simulink model "Supervisory_Logic"  (R2023b)
settings: Solver=FixedStepDiscrete  StartTime=0.0  StopTime=10  RelTol=1e-3
model workspace (MAT data in the model file):
  TsModel = 0.1
settings Model: ExtModeTrigDuration=8  Creator=vivekr  LastModifiedBy=vlenzi
settings SolverCC: AlgebraicLoopSolver=TrustRegion
settings DataIOCC: SaveFormat=StructureWithTime  SaveOutput=off  SignalLogging=off  DSMLogging=off  SaveTime=off  SignalLoggingName=logsOut
settings OptimizationCC: DefaultParameterBehavior=Inlined  UseDivisionForNetSlopeComputation=UseDivisionForReciprocalsOfIntegersOnly  ReuseModelBlockBuffer=off  EnhancedBackFolding=on  BooleansAsBitfields=on  PassReuseOutputArgsAs=Individual arguments  ExpressionDepthLimit=2147483647  StateBitsets=on  DataBitsets=on  ZeroExternalMemoryAtStartup=off  NoFixptDivByZeroProtection=on  EfficientFloat2IntCast=on  LifeSpan=1  MaxStackSize=64  SimCompilerOptimization=on  EfficientTunableParamExpr=on
settings DebuggingCC: ReadBeforeWriteMsg=DisableAll  WriteAfterWriteMsg=DisableAll  WriteAfterReadMsg=DisableAll  CheckExecutionContextPreStartOutputMsg=on  ParameterPrecisionLossMsg=none  UnconnectedInputMsg=warning  UnconnectedOutputMsg=warning  UnconnectedLineMsg=warning  UniqueDataStoreMsg=error  AllowSymbolicDim=off  ModelReferenceSymbolNameMessage=none  StateNameClashWarn=warning  StrictBusMsg=ErrorOnBusTreatedAsVector  SymbolicDimsDataTypeCodeGenerationDiagnostic=none  SFUnexpectedBacktrackingDiag=warning  SFNoUnconditionalDefaultTransitionDiag=warning  SFExecutionAtInitializationDiag=none  ArithmeticOperatorsInVariantConditions=warning
settings HardwareCC: TargetHWDeviceType=Generic->32-bit Embedded Processor
settings ModelReferenceCC: EnableRefExpFcnMdlSchedulingChecks=on  CheckModelReferenceTargetMessage=none  PropagateSignalLabelsOutOfModel=off
settings SFSimCC: SimUseLocalCustomCode=off  MATLABDynamicMemAlloc=off
settings RTWCC: Description=Embedded Coder  SystemTargetFile=ert.tlc  TemplateMakefile=ert_default_tmf  GenerateReport=on  RTWVerbose=off  RTWUseLocalCustomCode=off  IncludeHyperlinkInReport=on  PortableWordSizes=on  CodeExecutionProfiling=on  CodeProfilingSaveOptions=AllData  CodeProfilingInstrumentation=coarse  GenerateTraceInfo=on  GenerateTraceReport=on  GenerateTraceReportSl=on  GenerateTraceReportSf=on  GenerateTraceReportEml=on  GenerateCodeMetricsReport=on  DLArmComputeVersion=19.05
settings CodeAppCC: ForceParamTrailComments=on  IgnoreCustomStorageClasses=off  SimulinkDataObjDesc=on  CustomSymbolStrGlobalVar=rt$N$M  CustomSymbolStrType=$N$M  CustomSymbolStrFcn=$N$M$F  CustomSymbolStrMacro=$N$M  InsertBlockDesc=on  StateflowObjectComments=on  InternalIdentifier=Classic
settings ERTTargetCC: UtilityFuncGeneration=Shared location  MultiwordLength=2048  IncludeMdlTerminateFcn=off  CombineSignalStateStructs=on  SupportNonFinite=off  SupportComplex=off  ExtModeStaticAllocSize=2048  ERTCustomFileTemplate=example_file_process.tlc  ERTFilePackagingFormat=CompactWithDataFile  ConvertIfToSwitch=off  SuppressUnreachableDefaultCases=off
settings ConfigComp: CovMetricSettings=dw  CovSaveCumulativeToWorkspaceVar=on  CovSaveSingleToWorkspaceVar=on  CovExternalEMLEnable=off  CovSFcnEnable=off  PLC_TargetIDE=codesys35  PLC_MultiTBSigbuilderTimeRange=off  PLC_GenerateReusableCode=on  PLC_FoldFBCallOutputVar=on  PLC_RemoveUnusedSSMethodCallArguments=on  PLC_FBUseSubsystemInstanceName=on  PLC_UseCallOutputArgSyntax=off  PLC_EnableUnsignedAndDoubleTypes=off  PLC_EnableUDTSplitting=off  PLC_MaxFieldsInUDT=500  PLC_GenerateEnumSymbolicName=on  PLC_GenerateEnumCastFunction=on  PLC_InlineEnumCastFunction=on  PLC_GenerateWebView=on

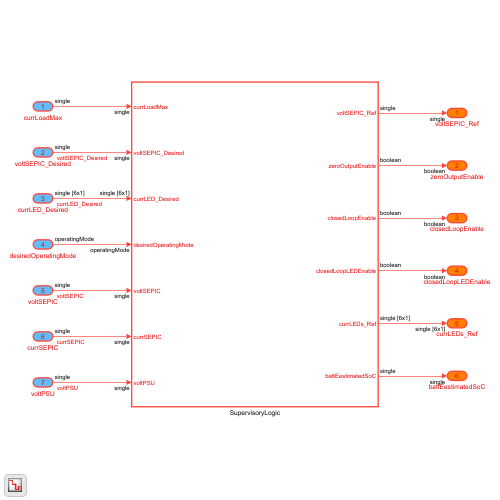
[thumbnail: Simulink's stored preview of the top-level diagram]
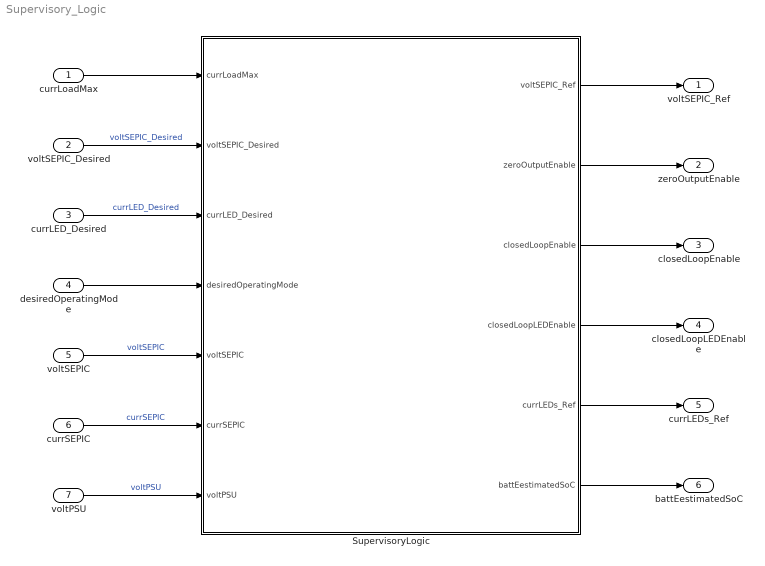
== system Supervisory_Logic ==
  currLoadMax : Inport  OutDataTypeStr=single  PortDimensions=1  SampleTime=TsModel
  voltSEPIC_Desired : Inport  Port=2  OutDataTypeStr=single  PortDimensions=1  SampleTime=TsModel
  currLED_Desired : Inport  Port=3  OutDataTypeStr=single  Unit=mA  PortDimensions=[6 1]  SampleTime=TsModel
  desiredOperatingMode : Inport  Port=4  OutDataTypeStr=Enum:operatingMode  PortDimensions=1  SampleTime=TsModel
  voltSEPIC : Inport  Port=5  OutDataTypeStr=single  Unit=V  PortDimensions=1  SampleTime=TsModel
  currSEPIC : Inport  Port=6  OutDataTypeStr=single  Unit=mA  PortDimensions=1  SampleTime=TsModel
  voltPSU : Inport  Port=7  OutDataTypeStr=single  Unit=V  PortDimensions=1  SampleTime=TsModel
  SupervisoryLogic : Subsystem  TreatAsAtomicUnit=on
      settings: RTWFcnNameOpts=Use subsystem name
  voltSEPIC_Ref : Outport  OutDataTypeStr=single  Unit=V  PortDimensions=1  SampleTime=TsModel
  zeroOutputEnable : Outport  Port=2  OutDataTypeStr=boolean  Unit=1  PortDimensions=1  SampleTime=TsModel
  closedLoopEnable : Outport  Port=3  OutDataTypeStr=boolean  Unit=1  PortDimensions=1  SampleTime=TsModel
  closedLoopLEDEnable : Outport  Port=4  OutDataTypeStr=boolean  Unit=1  PortDimensions=1  SampleTime=TsModel
  currLEDs_Ref : Outport  Port=5  OutDataTypeStr=single  Unit=mA  PortDimensions=[6 1 ]  SampleTime=TsModel
  battEestimatedSoC : Outport  Port=6  OutDataTypeStr=single  PortDimensions=1  SampleTime=TsModel
  wires:
  currLoadMax/1 -> SupervisoryLogic/1(currLoadMax)
  SupervisoryLogic/6(battEestimatedSoC) -> battEestimatedSoC/1
  SupervisoryLogic/5(currLEDs_Ref) -> currLEDs_Ref/1
  SupervisoryLogic/4(closedLoopLEDEnable) -> closedLoopLEDEnable/1
  voltPSU/1 -> SupervisoryLogic/7(voltPSU)  "voltPSU"
  voltSEPIC_Desired/1 -> SupervisoryLogic/2(voltSEPIC_Desired)  "voltSEPIC_Desired"
  currLED_Desired/1 -> SupervisoryLogic/3(currLED_Desired)  "currLED_Desired"
  SupervisoryLogic/3(closedLoopEnable) -> closedLoopEnable/1
  SupervisoryLogic/2(zeroOutputEnable) -> zeroOutputEnable/1
  SupervisoryLogic/1(voltSEPIC_Ref) -> voltSEPIC_Ref/1
  desiredOperatingMode/1 -> SupervisoryLogic/4(desiredOperatingMode)
  voltSEPIC/1 -> SupervisoryLogic/5(voltSEPIC)  "voltSEPIC"
  currSEPIC/1 -> SupervisoryLogic/6(currSEPIC)  "currSEPIC"

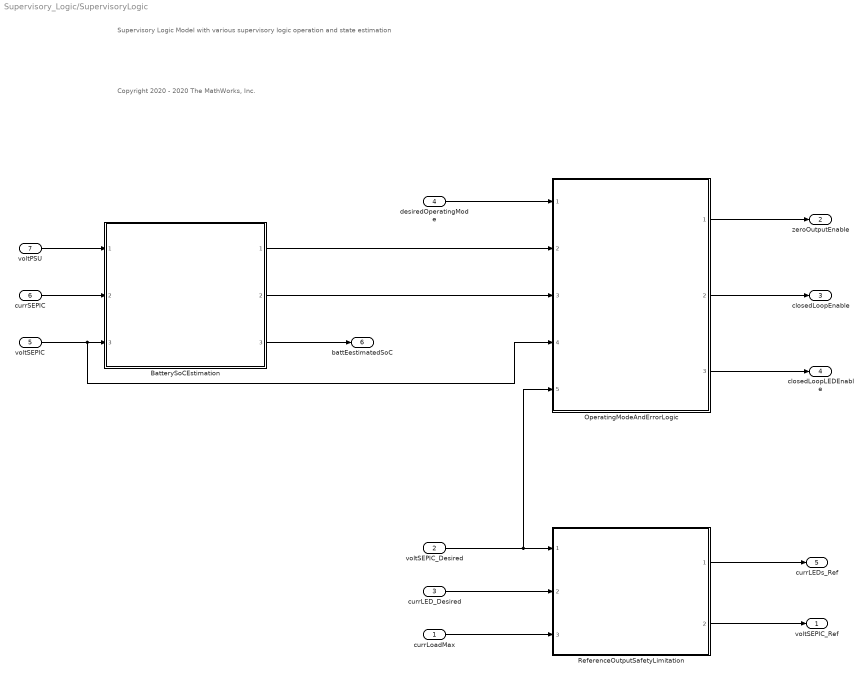
== system Supervisory_Logic/SupervisoryLogic ==
  note: Supervisory Logic
      | Model with various supervisory logic operation and state estimation
  note: Copyright 2020 - 2020 The MathWorks, Inc.
  currLoadMax : Inport  OutDataTypeStr=single  PortDimensions=1  SampleTime=TsModel
  voltSEPIC_Desired : Inport  Port=2  OutDataTypeStr=single  PortDimensions=1  SampleTime=TsModel
  currLED_Desired : Inport  Port=3  OutDataTypeStr=single  Unit=mA  PortDimensions=[6 1]  SampleTime=TsModel
  desiredOperatingMode : Inport  Port=4  OutDataTypeStr=Enum: operatingMode  PortDimensions=1  SampleTime=TsModel
  voltSEPIC : Inport  Port=5  OutDataTypeStr=single  Unit=V  PortDimensions=1  SampleTime=TsModel
  currSEPIC : Inport  Port=6  OutDataTypeStr=single  Unit=mA  PortDimensions=1  SampleTime=TsModel
  voltPSU : Inport  Port=7  OutDataTypeStr=single  Unit=V  PortDimensions=1  SampleTime=TsModel
  "BatterySoCEstimation " : Subsystem  TreatAsAtomicUnit=on  ReferencedSubsystem=BatterySoCEstimation
  OperatingModeAndErrorLogic : Subsystem  TreatAsAtomicUnit=on  ReferencedSubsystem=OperatingModeAndErrorLogic
  ReferenceOutputSafetyLimitation : Subsystem  TreatAsAtomicUnit=on  ReferencedSubsystem=ReferenceOutputSafetyLimitation
  voltSEPIC_Ref : Outport  OutDataTypeStr=single  Unit=V  PortDimensions=1  SampleTime=TsModel
  zeroOutputEnable : Outport  Port=2  OutDataTypeStr=boolean  Unit=1  PortDimensions=1  SampleTime=TsModel
  closedLoopEnable : Outport  Port=3  OutDataTypeStr=boolean  Unit=1  PortDimensions=1  SampleTime=TsModel
  closedLoopLEDEnable : Outport  Port=4  OutDataTypeStr=boolean  Unit=1  PortDimensions=1  SampleTime=TsModel
  currLEDs_Ref : Outport  Port=5  OutDataTypeStr=single  Unit=mA  PortDimensions=[6 1 ]  SampleTime=TsModel
  battEestimatedSoC : Outport  Port=6  OutDataTypeStr=single  PortDimensions=1  SampleTime=TsModel
  wires:
  OperatingModeAndErrorLogic/3 -> closedLoopLEDEnable/1
  voltSEPIC/1 -> "BatterySoCEstimation "/3, OperatingModeAndErrorLogic/4
  voltSEPIC_Desired/1 -> OperatingModeAndErrorLogic/5, ReferenceOutputSafetyLimitation/1
  currLoadMax/1 -> ReferenceOutputSafetyLimitation/3
  ReferenceOutputSafetyLimitation/1 -> currLEDs_Ref/1
  desiredOperatingMode/1 -> OperatingModeAndErrorLogic/1
  currLED_Desired/1 -> ReferenceOutputSafetyLimitation/2
  OperatingModeAndErrorLogic/1 -> zeroOutputEnable/1
  ReferenceOutputSafetyLimitation/2 -> voltSEPIC_Ref/1
  OperatingModeAndErrorLogic/2 -> closedLoopEnable/1
  voltPSU/1 -> "BatterySoCEstimation "/1
  currSEPIC/1 -> "BatterySoCEstimation "/2
  "BatterySoCEstimation "/1 -> OperatingModeAndErrorLogic/2
  "BatterySoCEstimation "/2 -> OperatingModeAndErrorLogic/3
  "BatterySoCEstimation "/3 -> battEestimatedSoC/1
